simulink model "slexHARFixedPointDeployExample"  (R2021a)
settings: Solver=FixedStepAuto  StartTime=0.0  StopTime=inf  RelTol=1e-3  EnableMultiTasking=on
PreLoadFcn:
  | % Pre-processing parameters
  | s = [1.0000   -1.0000         0    1.0000   -0.9004         0
  |     1.0000   -1.9996    1.0000    1.0000   -1.9203    0.9254
  |     1.0000   -1.9990    1.0000    1.0000   -1.9762    0.9791
  |     1.0000   -1.9986    1.0000    1.0000   -1.9929    0.9953];
  | 
  | fs = 10;
  | g = 0.9013;
  | featsDT = single(1);
  | lags = (0:32)';
  | tc = (1/fs)*lags;
undefined symbols (not defined in the file or in its folder): dfilt
libraries: microbitledlib x6, dspstat3 x3, microbitaccellib x1, statsLibrary x1, dsparch4 x1, dspsigops x1
settings Model: FPTShortcutValueString='{{},{''BaselineRun'',1,1,1,''BaselineRun'','''',{},''M'','''',''''},{''EmbeddedRun'',1,1,1,''EmbeddedRun'','''',{},''M'','''',''''},{''EmbeddedRun_2'',1,1,1,''EmbeddedRun_2'','''',{},''M'','''',''''}}'  SILPILModeSetting=veronly  ExtModeTrigDuration=5  Creator=The MathWorks, Inc.  LastModifiedBy=The MathWorks, Inc.
settings SolverCC: AlgebraicLoopSolver=TrustRegion
settings DataIOCC: ExternalInput=ts
settings OptimizationCC: EnhancedBackFolding=on  PassReuseOutputArgsAs=Individual arguments  ZeroExternalMemoryAtStartup=off  ZeroInternalMemoryAtStartup=off  MaxStackSize=64  OptimizeBlockOrder=speed  DifferentSizesBufferReuse=on  OptimizationCustomize=off  EfficientTunableParamExpr=on
settings DebuggingCC: SignalRangeChecking=warning  ParameterTunabilityLossMsg=error  SFMachineParentedDataDiag=warning
settings HardwareCC: ProdBitPerPointer=32  ProdBitPerSizeT=32  ProdBitPerPtrDiffT=32  ProdLargestAtomicInteger=Long  ProdLargestAtomicFloat=Double  ProdWordSize=32  ProdHWDeviceType=ARM Compatible->ARM Cortex
settings SFSimCC: MATLABDynamicMemAlloc=off
settings RTWCC: SystemTargetFile=ert.tlc  HardwareBoard=BBC micro:bit  TemplateMakefile=ert_default_tmf  GenerateReport=on  Toolchain=GNU Tools for ARM Embedded Processors  BuildConfiguration=Faster Runs  LaunchReport=on  GenerateCodeMetricsReport=on
settings CodeAppCC: ForceParamTrailComments=on  IgnoreCustomStorageClasses=off  OperatorAnnotations=on  SimulinkDataObjDesc=on  SFDataObjDesc=on  InsertBlockDesc=on
settings ERTTargetCC: SupportComplex=off  SupportContinuousTime=on  SupportVariableSizeSignals=on  ExtModeStaticAllocSize=65536

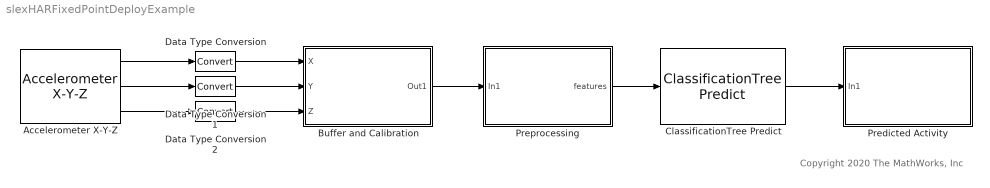
== system slexHARFixedPointDeployExample ==
  note: Copyright 2020 The MathWorks, Inc
  Accelerometer X-Y-Z : microbitaccellib/Accelerometer X-Y-Z  ODR=800Hz  Accelfullrange=-4g to +4g  SampleTime=-1
      settings: SourceProductBaseCode=MICROBIT
  Buffer and Calibration : Subsystem
  ClassificationTree Predict : statsLibrary/Classification/ClassificationTree Predict  TrainedLearner=classificationTree  ShowOutputScore=off  LabelDataTypeStr=Inherit: Inherit via back propagation  LabelOutMin=[]  LabelOutMax=[]  ScoreOutMin=[]  ScoreOutMax=[]  RawScoreOutMin=[]  RawScoreOutMax=[]  StoredEnumName=treeMdl_enumLabels
      settings: SourceProductBaseCode=ST
  Data Type Conversion : DataTypeConversion
  Data Type Conversion1 : DataTypeConversion
  Data Type Conversion2 : DataTypeConversion
  Predicted Activity : Subsystem
  Preprocessing : Subsystem
  wires:
  ClassificationTree Predict/1 -> Predicted Activity/1(In1)
  Accelerometer X-Y-Z/1 -> Data Type Conversion/1
  Accelerometer X-Y-Z/2 -> Data Type Conversion1/1
  Accelerometer X-Y-Z/3 -> Data Type Conversion2/1
  Data Type Conversion/1 -> Buffer and Calibration/1(X)
  Data Type Conversion2/1 -> Buffer and Calibration/3(Z)
  Preprocessing/1(features) -> ClassificationTree Predict/1
  Buffer and Calibration/1(Out1) -> Preprocessing/1(In1)
  Data Type Conversion1/1 -> Buffer and Calibration/2(Y)

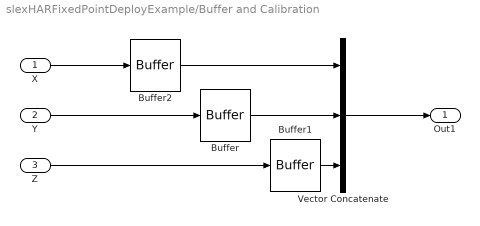
== system slexHARFixedPointDeployExample/Buffer and Calibration ==
  X : Inport  OutDataTypeStr=fixdt(1,16,10)
  Y : Inport  Port=2  OutDataTypeStr=fixdt(1,16,10)
  Z : Inport  Port=3  OutDataTypeStr=fixdt(1,16,10)
  Buffer : Buffer  N=32  V=12  OutputFrames=off
  Buffer1 : Buffer  N=32  V=12  OutputFrames=off
  Buffer2 : Buffer  N=32  V=12  OutputFrames=off
  Vector Concatenate : Concatenate  NumInputs=3  Mode=Multidimensional array  ConcatenateDimension=2
  Out1 : Outport
  wires:
  Buffer1/1 -> Vector Concatenate/3
  Buffer2/1 -> Vector Concatenate/1
  Z/1 -> Buffer1/1
  Buffer/1 -> Vector Concatenate/2
  Vector Concatenate/1 -> Out1/1
  X/1 -> Buffer2/1
  Y/1 -> Buffer/1

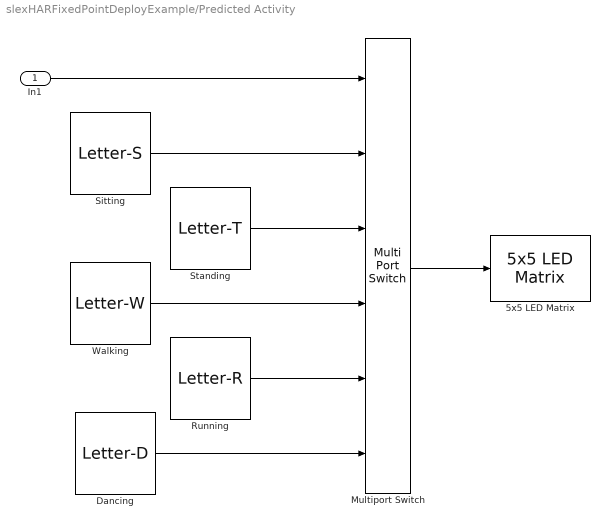
== system slexHARFixedPointDeployExample/Predicted Activity ==
  In1 : Inport
  5x5 LED Matrix : microbitledlib/5x5 LED Matrix  LED_mat=[0 1 1 1 0;1 0 1 0 1;1 1 0 1 1; 1 0 1 0 1;0 1 1 1 0]
      settings: SourceProductBaseCode=MICROBIT
  Dancing : microbitledlib/LED Images/Letter-D  L00=on  L01=on  L02=on  L03=off  L04=off  L10=on  L11=off  L12=off  L13=on  L14=off  L20=on  L21=off  L22=off  L23=on  L24=off  L30=on  L31=off  L32=off  L33=on  L34=off  L40=on  L41=on  L42=on  L43=off  L44=off
      settings: SourceProductBaseCode=MICROBIT
  Multiport Switch : MultiPortSwitch  Inputs=5
  Running : microbitledlib/LED Images/Letter-R  L00=on  L01=on  L02=on  L03=off  L04=off  L10=on  L11=off  L12=off  L13=on  L14=off  L20=on  L21=on  L22=on  L23=off  L24=off  L30=on  L31=off  L32=off  L33=on  L34=off  L40=on  L41=off  L42=off  L43=off  L44=on
      settings: SourceProductBaseCode=MICROBIT
  Sitting : microbitledlib/LED Images/Letter-S  L00=off  L01=on  L02=on  L03=on  L04=off  L10=on  L11=off  L12=off  L13=off  L14=off  L20=off  L21=on  L22=on  L23=off  L24=off  L30=off  L31=off  L32=off  L33=on  L34=off  L40=on  L41=on  L42=on  L43=off  L44=off
      settings: SourceProductBaseCode=MICROBIT
  Standing : microbitledlib/LED Images/Letter-T  L00=on  L01=on  L02=on  L03=on  L04=on  L10=off  L11=off  L12=on  L13=off  L14=off  L20=off  L21=off  L22=on  L23=off  L24=off  L30=off  L31=off  L32=on  L33=off  L34=off  L40=off  L41=off  L42=on  L43=off  L44=off
      settings: SourceProductBaseCode=MICROBIT
  Walking : microbitledlib/LED Images/Letter-W  L00=on  L01=off  L02=off  L03=off  L04=on  L10=on  L11=off  L12=off  L13=off  L14=on  L20=on  L21=off  L22=on  L23=off  L24=on  L30=on  L31=on  L32=off  L33=on  L34=on  L40=on  L41=off  L42=off  L43=off  L44=on
      settings: SourceProductBaseCode=MICROBIT
  wires:
  In1/1 -> Multiport Switch/1
  Sitting/1 -> Multiport Switch/2
  Standing/1 -> Multiport Switch/3
  Walking/1 -> Multiport Switch/4
  Running/1 -> Multiport Switch/5
  Dancing/1 -> Multiport Switch/6
  Multiport Switch/1 -> 5x5 LED Matrix/1

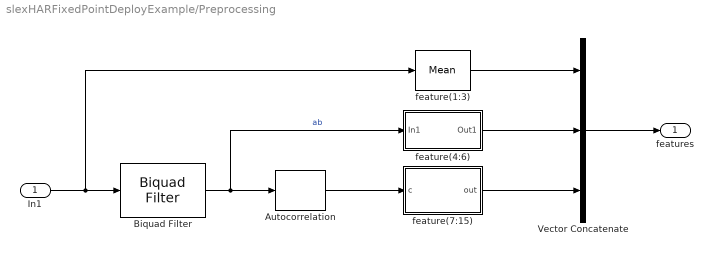
== system slexHARFixedPointDeployExample/Preprocessing ==
  In1 : Inport  OutDataTypeStr=fixdt(1,16,10)
  Autocorrelation : dspstat3/Autocorrelation  AllPositiveLags=on  maxlag=1  bias=None  domain=Time  roundingMode=Floor  overflowMode=off  accumMode=Binary point scaling  accumWordLength=32  accumFracLength=24  accumDataTypeStr=fixdt([],32,24)  accumLastDataTypeStr=fixdt([],32,24)  outputMode=Binary point scaling  outputWordLength=16  outputFracLength=10  outputDataTypeStr=fixdt([],16,10)  outputMin=[]  outputMax=[]  outputLastDataTypeStr=fixdt([],16,10)
      settings: SourceProductBaseCode=DS
  Biquad Filter : dsparch4/Biquad Filter  FilterSource=Dialog parameters  CoeffSource=Specify via dialog  FilterObject=dfilt.df2tsos([1 0.3 0.4],[1 0.1 0.2])  IIRFiltStruct=Direct form II transposed  BiQuadCoeffs=s  ScaleValues=g  IC=0  ICnum=0  ICden=0  a0Flag=Warning  optimizeScaleValues=on  ScaleValueMode=Specify via input port (g)  roundingMode=Floor  overflowMode=off  scaleValueFracLength=14  denProdOutputFracLength=30  denAccumFracLength=30  secondMemoryFracLength=15  outputMode=Binary point scaling  outputWordLength=16  outputFracLength=14
  Vector Concatenate : Concatenate  NumInputs=3
  feature(1:3) : dspstat3/Mean  run=off  InputProcessing=Columns as channels (frame based)  reset_popup=None  directionMode=Each column  dimension=1  roiEnable=off  roiType=Rectangles  roiPortion=Entire ROI  roiOutput=Individual statistics for each ROI  roiFlag=off  roundingMode=Floor  overflowMode=off  outputMode=Binary point scaling  outputWordLength=16  outputFracLength=10  outputDataTypeStr=fixdt([],16,10)  outputMin=[]  outputMax=[]  outputLastDataTypeStr=fixdt([],16,10)
  feature(4:6) : Subsystem  Tag=DecoupledSystem
  feature(7:15) : Subsystem
  features : Outport
  wires:
  In1/1 -> feature(1:3)/1, Biquad Filter/1
  Biquad Filter/1 -> feature(4:6)/1(In1), Autocorrelation/1  "ab"
  Autocorrelation/1 -> feature(7:15)/1(c)
  feature(1:3)/1 -> Vector Concatenate/1
  feature(4:6)/1(Out1) -> Vector Concatenate/2
  feature(7:15)/1(out) -> Vector Concatenate/3
  Vector Concatenate/1 -> features/1

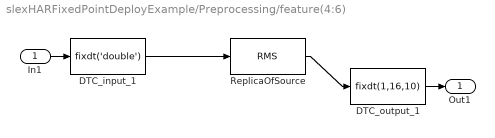
== system slexHARFixedPointDeployExample/Preprocessing/feature(4:6) ==
  In1 : Inport  LockScale=on
  DTC_input_1 : DataTypeConversion  OutDataTypeStr=fixdt('double')  RndMeth=Nearest  LockScale=on
  DTC_output_1 : DataTypeConversion  OutDataTypeStr=fixdt(1,16,10)
  ReplicaOfSource : dspstat3/RMS  run=off  directionMode=Each column  dimension=1  InputProcessing=Columns as channels (frame based)  reset_popup=None
  Out1 : Outport  LockScale=on
  wires:
  In1/1 -> DTC_input_1/1
  DTC_output_1/1 -> Out1/1
  ReplicaOfSource/1 -> DTC_output_1/1
  DTC_input_1/1 -> ReplicaOfSource/1

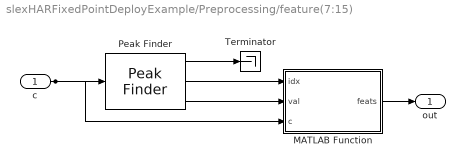
== system slexHARFixedPointDeployExample/Preprocessing/feature(7:15) ==
  c : Inport  OutDataTypeStr=fixdt(1,16,10)
  MATLAB Function : Subsystem  TreatAsAtomicUnit=on  Variant=on  VariantControlMode=label  VariantControl=Choice  LabelModeActiveChoice=(default)
  Peak Finder : dspsigops/Peak Finder  polarity=Maxima  indexBase=One  outputIdx=on  outputVal=on  maxPeaks=10  NoiseDistinguish=on  thresh=0.0005  roundingMode=Floor  overflowMode=off
      settings: SourceProductBaseCode=DS  allowOverrides=off
  Terminator : Terminator
  out : Outport
  wires:
  c/1 -> Peak Finder/1, MATLAB Function/3(c)
  Peak Finder/1 -> Terminator/1
  Peak Finder/2 -> MATLAB Function/1(idx)
  Peak Finder/3 -> MATLAB Function/2(val)
  MATLAB Function/1(feats) -> out/1

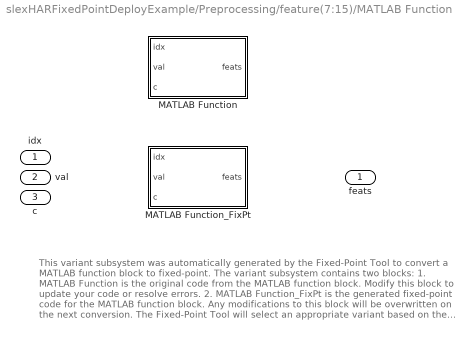
== system slexHARFixedPointDeployExample/Preprocessing/feature(7:15)/MATLAB Function ==
  note: This variant subsystem was automatically generated by the Fixed-Point Tool to convert a MATLAB function block to fixed-point.
      |
      | The variant subsystem contains two blocks:
      | 1. MATLAB Function is the original code from the MATLAB function block. Modify this block to update your code or resolve errors.
      |
      | 2. MATLAB Function_FixPt is the generated fixed-point code for the MATLAB function block. Any modifications to this block will be overwritten on the next conversion.
      |
      | The Fixed-Point Tool will select an appropriate variant based on the Model Settings. Learn more. .
  idx : Inport
  val : Inport  Port=2
  c : Inport  Port=3
  MATLAB Function : MATLAB Function  TreatAsAtomicUnit=on  VariantControl=false()
  MATLAB Function_FixPt : MATLAB Function  TreatAsAtomicUnit=on  VariantControl=(default)
  feats : Outport

== matlab function slexHARFixedPointDeployExample/Preprocessing/feature(7:15)/MATLAB Function/MATLAB Function_FixPt ==
  settings: fimath=fimath('RoundingMethod', 'Floor', 'OverflowAction', 'Wrap', 'ProductMode', 'FullPrecision', 'MaxProductWordLength', 128, 'SumMode', 'FullPrecision', 'MaxSumWordLength', 128)
  data: idx input; val input; c input; feats output; tc parameter
%auto-generated
%#codegen
function feats = fcn_fixpt(idx,val,c,tc)
fm = get_fimath();
c = fi(c, 1, 16, 10, fm);
idx = fi(idx, 0, 32, 27, fm);
tc = fi(tc, 0, 16, 14, fm);
val = fi(val, 1, 16, 10, fm);

feats = fi(zeros(9,1,'like',val), 1, 16, 10, fm);
for k = 1:3
%     [pks,locs] = findpeaks([0;c(:,k)],...
%         'minpeakprominence',minprom,...
%         'minpeakdistance',minpkdist);
    nzInds = idx(:,k)>fi(0, 0, 1, 0, fm);
    locs = fi(idx(nzInds,k), 0, 32, 27, fm);
    pks = fi(val(nzInds,k), 1, 16, 10, fm);
    
    tcl = fi(tc(locs), 0, 16, 14, fm);

    % Feature 1 - peak height at 0
    feats(3*(k-1)+1) = c(1,k);
    % Features 2 and 3 - position and height of first peak 
    if(length(tcl) >= 2)   % else f2,f3 already 0
        feats(3*(k-1)+2) = tcl(2);
        feats(3*(k-1)+3) = pks(2);
    end
end
end


function fm = get_fimath()
	fm = fimath('RoundingMethod', 'Floor',...
	     'OverflowAction', 'Wrap',...
	     'ProductMode','FullPrecision',...
	     'MaxProductWordLength', 128,...
	     'SumMode','FullPrecision',...
	     'MaxSumWordLength', 128);
end

== matlab function slexHARFixedPointDeployExample/Preprocessing/feature(7:15)/MATLAB Function/MATLAB Function ==
  data: idx input; val input; c input; feats output; tc parameter
function feats = fcn(idx,val,c,tc)
feats = zeros(9,1,'like',val);
for k = 1:3
%     [pks,locs] = findpeaks([0;c(:,k)],...
%         'minpeakprominence',minprom,...
%         'minpeakdistance',minpkdist);
    nzInds = idx(:,k)>0;
    locs = idx(nzInds,k);
    pks = val(nzInds,k);
    
    tcl = tc(locs);

    % Feature 1 - peak height at 0
    feats(3*(k-1)+1) = c(1,k);
    % Features 2 and 3 - position and height of first peak 
    if(length(tcl) >= 2)   % else f2,f3 already 0
        feats(3*(k-1)+2) = tcl(2);
        feats(3*(k-1)+3) = pks(2);
    end
end
